simulink model "PVTOL_SMC_Asintotico"  (R2026b)
settings Model: Creator=nestorhernandezcastellanos  LastModifiedBy=nestorhernandezcastellanos

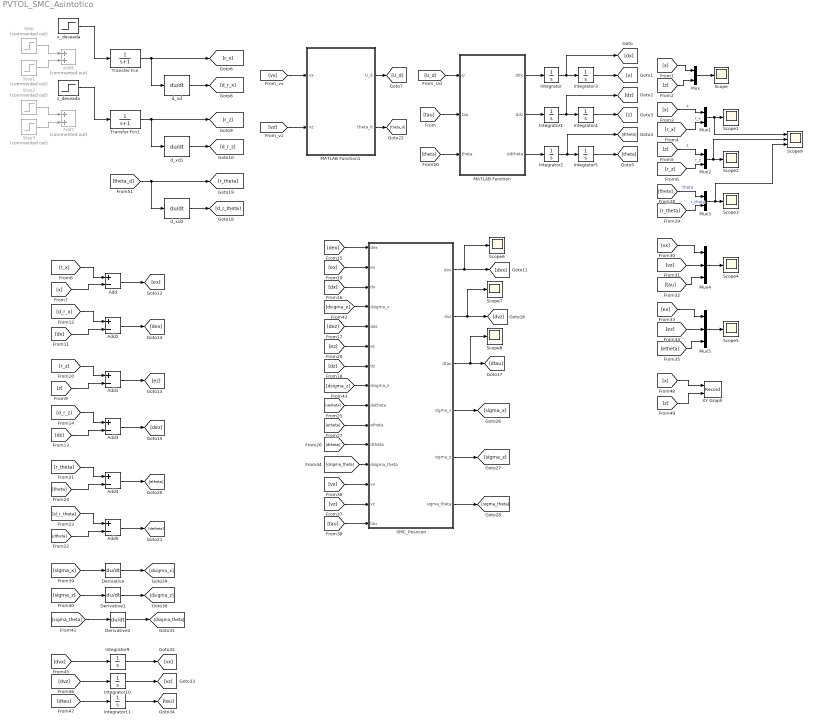
== system PVTOL_SMC_Asintotico ==
  Add{,1..5} (6 alike) : Sum  Inputs=+-
  Add6 : Sum  Commented=on
  Add7 : Sum  Commented=on
  Derivative : Derivative
  Derivative1 : Derivative
  Derivative2 : Derivative
  Integrator{,1..5,9..11} (9 alike) : Integrator
  MATLAB Function : MATLAB Function  TreatAsAtomicUnit=on
  MATLAB Function1 : MATLAB Function  TreatAsAtomicUnit=on
  Mux{,1..3} (4 alike) : Mux  Inputs=2
  Mux4 : Mux  Inputs=3
  Mux5 : Mux  Inputs=3
  SMC_Posicion : MATLAB Function  TreatAsAtomicUnit=on
  Scope{,1..8} (9 alike) : Scope
      Scope settings: ActiveDisplayYMinimum=1.7015017403321495  ActiveDisplayYMaximum=4.686484337010655
      Scope1 settings: ActiveDisplayYMinimum=-0.62499999649831228  ActiveDisplayYMaximum=5.6249999684848113
      Scope2 settings: ActiveDisplayYMinimum=-0.62499999649831228  ActiveDisplayYMaximum=5.6249999684848113  DataLoggingVariableName=ScopeData2
      Scope3 settings: ActiveDisplayYMinimum=-0.62499999649831228  ActiveDisplayYMaximum=5.6249999684848113  DataLoggingVariableName=ScopeData3
      Scope4 settings: ActiveDisplayYMinimum=-1.450142493908271  ActiveDisplayYMaximum=1.4786584506258409  DataLoggingVariableName=ScopeData4
      Scope5 settings: ActiveDisplayYMinimum=-0.41525140644879627  ActiveDisplayYMaximum=3.7372626580391675  DataLoggingVariableName=ScopeData5
      Scope6 settings: ActiveDisplayYMinimum=-375.96530288775057  ActiveDisplayYMaximum=375.89482808407041  DataLoggingVariableName=ScopeData6
      Scope7 settings: ActiveDisplayYMinimum=-375.96530288775057  ActiveDisplayYMaximum=375.89482808407041  DataLoggingVariableName=ScopeData7
      Scope8 settings: ActiveDisplayYMinimum=-375.96530288775057  ActiveDisplayYMaximum=375.89482808407041  DataLoggingVariableName=ScopeData8
  Scope9 : Scope  NumInputPorts=3
      settings: ActiveDisplayYMinimum=-0.65641521642220824  ActiveDisplayYMaximum=5.9077369477998749  DataLoggingVariableName=ScopeData9
  Step : Step  Commented=on  FinalValue=3  SampleTime=0
  Step1 : Step  Commented=on  Time=15  FinalValue=7  SampleTime=0
  Step2 : Step  Commented=on  FinalValue=3  SampleTime=0
  Step3 : Step  Commented=on  Time=15  FinalValue=7  SampleTime=0
  Transfer Fcn : TransferFcn  Denominator=[1 1]
  Transfer Fcn1 : TransferFcn  Denominator=[1 1]
  XY Graph : Record  NumPorts=2.0  FileSettingsInternal="{\"entries\":[{\"content\":{\"excelSettings\":{\"content\":{},\"type\":\"Streamout.ExcelSettings\"},\"parquetSettings\":{\"content\":{},\"type\":\"Streamout.ParquetSettings\"}},\"type\":\"Streamout.FileSettingStorage\",\"uuid\":\"\"}],\"packageUris\":[\"http:\\/\\/schema.mathworks.com\\/mf0\\/streamout_blocks\\/R2020a\"],\"version\":\"1.0\"}"  FrameSettings=[0, 0]  Layout=[1 1]  SignalsInternal="{\"entries\":[{\"content\":{\"signals\":[{\"content\":{\"blockPath\":[],\"dimensions\":[1],\"domain\":\"\",\"lineColor\":\"#a2142f\",\"plots\":[ 1 ],\"port\":1,\"sid\":[\"\"],\"signalID\":1,\"signalName\":\"From48\"},\"type\":\"RecordBlkView.Signal\",\"uuid\":\"\"},{\"content\":{\"blockPath\":[],\"dimensions\":[1],\"domain\":\"\",\"lineColor\":\"#139fff\",\"plots\":[ 1 ],\"port\":2,\"sid\":[\"\"],\"signalID\":2,\"signalName\":\"From49\"},\"type\":\"RecordBlkView.Signal\",\"uuid\":\"\"}]},\"type\":\"RecordBlkView.InputSignals\",\"uuid\":\"\"}],\"packageUris\":[\"http:\\/\\/schema.mathworks.com\\/mf0\\/streamout_blocks\\/R2020a\"],\"version\":\"1.0\"}"  VisualizationBindings="{\"xyplotplugin\":{\"info\":[{\"series\":[{\"bindingParametersList\":[{\"parameter\":\"X-Axis\",\"signalID\":1,\"signalName\":\"From48\"},{\"parameter\":\"Y-Axis\",\"signalID\":2,\"signalName\":\"From49\"}],\"seriesID\":0}],\"subplotID\":1}]}}"  CompatibilityTag=XY
  d_xd : Derivative
  d_xd1 : Derivative
  d_xd2 : Derivative
  x_deseada : Step  FinalValue=5  SampleTime=0
  z_deseada : Step  FinalValue=5  SampleTime=0
  wires:
  Mux/1 -> Scope/1
  [z] -> Mux/2
  [x] -> Mux/1
  [x] -> Mux1/1  "x"
  [r_x] -> Mux1/2  "r_x"
  [r_z] -> Mux2/2  "r_z"
  [z] -> Mux2/1  "z"
  [r_x] -> Add/1
  [x] -> Add/2
  Add/1 -> [ex]
  [z] -> Add1/2
  [r_z] -> Add1/1
  Add2/1 -> [dex]
  [dx] -> Add2/2
  [d_r_x] -> Add2/1
  [d_r_z] -> Add3/1
  [dz] -> Add3/2
  Add3/1 -> [dez]
  SMC_Posicion/1(dvx) -> Scope6/1, [dvx]
  SMC_Posicion/2(dvz) -> Scope7/1, [dvz]
  SMC_Posicion/3(dtau) -> Scope8/1, [dtau]
  [dex] -> SMC_Posicion/1(dex)
  [dx] -> SMC_Posicion/3(dx)
  [dez] -> SMC_Posicion/5(dez)
  [dz] -> SMC_Posicion/7(dz)
  [ex] -> SMC_Posicion/2(ex)
  [ez] -> SMC_Posicion/6(ez)
  Add5/1 -> [detheta]
  [dtheta] -> Add5/2
  [d_r_theta] -> Add5/1
  [r_theta] -> Add4/1
  [theta] -> Add4/2
  [detheta] -> SMC_Posicion/9(detheta)
  [etheta] -> SMC_Posicion/10(etheta)
  [dtheta] -> SMC_Posicion/11(dtheta)
  [theta] -> Mux3/1  "theta"
  [r_theta] -> Mux3/2  "r_theta"
  Mux4/1 -> Scope4/1
  [vz] -> Mux4/2
  [vx] -> Mux4/1
  [tau] -> Mux4/3
  [etheta] -> Mux5/3
  [ex] -> Mux5/1
  [ez] -> Mux5/2
  Mux5/1 -> Scope5/1
  Add1/1 -> [ez]
  Add4/1 -> [etheta]
  SMC_Posicion/4(sigma_x) -> [sigma_x]
  SMC_Posicion/5(sigma_z) -> [sigma_z]
  SMC_Posicion/6(sigma_theta) -> [sigma_theta]
  [sigma_x] -> Derivative/1
  [sigma_z] -> Derivative1/1
  Derivative/1 -> [dsigma_x]
  Derivative1/1 -> [dsigma_z]
  Derivative2/1 -> [dsigma_theta]
  [sigma_theta] -> Derivative2/1
  [dsigma_x] -> SMC_Posicion/4(dsigma_x)
  [dsigma_z] -> SMC_Posicion/8(dsigma_z)
  [dsigma_theta] -> SMC_Posicion/12(dsigma_theta)
  [dvx] -> Integrator9/1
  [dvz] -> Integrator10/1
  [dtau] -> Integrator11/1
  Integrator9/1 -> [vx]
  Integrator10/1 -> [vz]
  Integrator11/1 -> [tau]
  [vx] -> SMC_Posicion/13(vx)
  [vz] -> SMC_Posicion/14(vz)
  [tau] -> SMC_Posicion/15(tau)
  [x] -> XY Graph/1
  [z] -> XY Graph/2
  x_deseada/1 -> Transfer Fcn/1
  [theta] -> MATLAB Function/3(theta)
  Integrator/1 -> [dx], Integrator3/1
  Transfer Fcn1/1 -> d_xd1/1, [r_z]
  Integrator5/1 -> [theta]
  [vx] -> MATLAB Function1/1(vx)
  MATLAB Function/1(ddx) -> Integrator/1
  d_xd/1 -> [d_r_x]
  MATLAB Function1/1(U_d) -> [U_d]
  [vz] -> MATLAB Function1/2(vz)
  MATLAB Function/2(ddz) -> Integrator1/1
  MATLAB Function1/2(theta_d) -> [theta_d]
  [tau] -> MATLAB Function/2(tau)
  [theta_d] -> [r_theta], d_xd2/1
  Integrator2/1 -> [dtheta], Integrator5/1
  d_xd1/1 -> [d_r_z]
  Integrator3/1 -> [x]
  d_xd2/1 -> [d_r_theta]
  MATLAB Function/3(ddtheta) -> Integrator2/1
  Step/1 -> Add6/1
  Integrator1/1 -> [dz], Integrator4/1
  Step1/1 -> Add6/2
  Transfer Fcn/1 -> [r_x], d_xd/1
  Step3/1 -> Add7/2
  z_deseada/1 -> Transfer Fcn1/1
  Step2/1 -> Add7/1
  Integrator4/1 -> [z]
  [U_d] -> MATLAB Function/1(U)
  Mux1/1 -> Scope9/1, Scope1/1
  Mux3/1 -> Scope9/3, Scope3/1
  Mux2/1 -> Scope9/2, Scope2/1

== matlab function PVTOL_SMC_Asintotico/MATLAB Function1 ==
  data: vx input; U_d output; vz input; theta_d output
function [U_d,theta_d] = linealizacion(vx,vz)

g = 9.81;                                  
U_d = sqrt(vx^2 + (vz+g)^2);                 
theta_d = atan2(-vx,vz+g);

== matlab function PVTOL_SMC_Asintotico/MATLAB Function ==
  data: U input; ddx output; tau input; theta input; ddz output; ddtheta output
function [ddx,ddz,ddtheta] = planta(U,tau,theta)

g = 9.81;                                       

ddx = -U*sin(theta);                            
ddz = U*cos(theta)-g;                           
ddtheta = tau;

== matlab function PVTOL_SMC_Asintotico/SMC_Posicion ==
  data: dex input; ex input; dx input; dsigma_x input; dez input; ez input; dz input; dsigma_z input; detheta input; etheta input; dtheta input; dsigma_theta input; vx input; dvx output; vz input; dvz output; dtau output; tau input; sigma_x output; sigma_z output; sigma_theta output
function [dvx, dvz, dtau, sigma_x, sigma_z, sigma_theta] = controlador(dex, ex, dx, dsigma_x, dez, ez, dz, dsigma_z, detheta, etheta, dtheta,dsigma_theta, vx, vz, tau)

% Parámetros del SMC asintótico
mx = 1.37;
msx = 9.5;
Kx = 20.5;

mz = 8;
msz = 1.5;
Kz = 2;

mtheta = 1.6;
mstheta = 25;
Ktheta = 25;

% Superficies principales
sigma_x = dex + mx*ex;
sigma_z = dez + mz*ez;
sigma_theta = detheta + mtheta*etheta;

% Superficies auxiliares
Sx = dsigma_x + msx*sigma_x;
Sz = dsigma_z + msz*sigma_z;
Stheta = dsigma_theta + mstheta*sigma_theta;

% Controladores dinámicos
dvx = -mx*msx*dx - (mx + msx)*vx + Kx*sign(Sx);
dvz = -mz*msz*dz - (mz + msz)*vz + Kz*sign(Sz);
dtau = -mtheta*mstheta*dtheta - (mtheta + mstheta)*tau + Ktheta*sign(Stheta);
